simulink model "xyzController"  (R2015b)
settings: Solver=ode45  StartTime=0.0  StopTime=100  RelTol=1e-3
values from neighbouring files (symbols this model uses):
  Kx = -kth*(w1_bar^2+w2_bar^2+w3_bar^2+w4_bar^2)    [xyzController.m]
  Ky = kth*(w1_bar^2+w2_bar^2+w3_bar^2+w4_bar^2)    [xyzController.m]
  Kz = -2*kth*w1_bar^2    [xyzController.m]
  m = 0.7    [Parameters.m]
undefined symbols (not defined in the file or in its folder): Cx, Cy, Cz
settings Model: Creator=Amalie  LastModifiedBy=USUARIO
settings DataIOCC: SaveFormat=Array
settings HardwareCC: ProdBitPerPointer=32  ProdLargestAtomicFloat=None  ProdIntDivRoundTo=Undefined  ProdEndianess=Unspecified  ProdWordSize=32  ProdHWDeviceType=32-bit Generic
settings GRTTargetCC: GeneratePreprocessorConditionals=Disable all
settings ConfigComp: CovModelRefEnable=Off

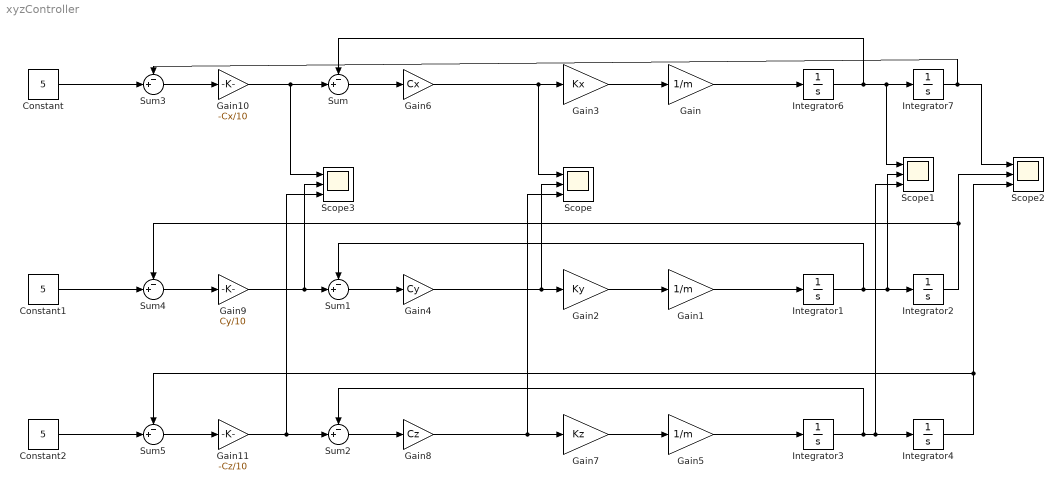
== system xyzController ==
  Constant : Constant  Value=5
  Constant1 : Constant  Value=5
  Constant2 : Constant  Value=5
  Gain : Gain  Gain=1/m
  Gain1 : Gain  Gain=1/m
  Gain10 : Gain  Gain=-Cx/10
  Gain11 : Gain  Gain=-Cz/10
  Gain2 : Gain  Gain=Ky
  Gain3 : Gain  Gain=Kx
  Gain4 : Gain  Gain=Cy
  Gain5 : Gain  Gain=1/m
  Gain6 : Gain  Gain=Cx
  Gain7 : Gain  Gain=Kz
  Gain8 : Gain  Gain=Cz
  Gain9 : Gain  Gain=Cy/10
  Integrator{1..4,6..7} (6 alike) : Integrator
  Scope{,1..3} (4 alike) : Scope  NumInputPorts=3
  Sum{,1..5} (6 alike) : Sum  Inputs=-+|
  wires:
  Gain/1 -> Integrator6/1
  Gain3/1 -> Gain/1
  Sum/1 -> Gain6/1
  Gain6/1 -> Scope/1, Gain3/1
  Gain1/1 -> Integrator1/1
  Gain2/1 -> Gain1/1
  Sum1/1 -> Gain4/1
  Gain4/1 -> Gain2/1, Scope/2
  Integrator6/1 -> Sum/1, Scope1/1, Integrator7/1
  Integrator1/1 -> Sum1/1, Integrator2/1, Scope1/2
  Gain5/1 -> Integrator3/1
  Gain7/1 -> Gain5/1
  Sum2/1 -> Gain8/1
  Gain8/1 -> Gain7/1, Scope/3
  Integrator3/1 -> Sum2/1, Integrator4/1, Scope1/3
  Sum3/1 -> Gain10/1
  Constant/1 -> Sum3/2
  Sum4/1 -> Gain9/1
  Constant1/1 -> Sum4/2
  Integrator7/1 -> Scope2/1, Sum3/1
  Integrator2/1 -> Sum4/1, Scope2/2
  Sum5/1 -> Gain11/1
  Constant2/1 -> Sum5/2
  Integrator4/1 -> Sum5/1, Scope2/3
  Gain10/1 -> Scope3/1, Sum/2
  Gain9/1 -> Scope3/2, Sum1/2
  Gain11/1 -> Scope3/3, Sum2/2
